simulink model "State_Flowc"  (R2017a)
settings: Solver=FixedStepDiscrete  StartTime=0.0  StopTime=inf  FixedStep=0.001  RelTol=1e-3  EnableMultiTasking=on
libraries: xpcethercatlib x31, simulink x4, simulink_extras x4, commutil2 x2
(part 2 of 2)

== matlab function State_Flowc/Movimento Braccia/Traiettorie figure/Quadrato ==
  data: xq output; yq output; t input; T input; h input; xq_p output; yq_p output
function [xq, yq, xq_p, yq_p] = Quadrato(t, T, h)
xv = 0.4;
xj = 0.1;
x1 = t/(0.5*T/4);
x2 = (t-0.5*T/4)/(T/4);
x3 = (t-1.5*T/4)/(T/4);
x4 = (t-2.5*T/4)/(T/4);
x5 = (t-3.5*T/4)/(0.5*T/4);
Ca = 1/((1-xv)*(xv-xj));
% Ca = 1/(xv*(1-xv));
% Cv = 1/(1-xv);


if t > 0 && t <= 0.5*T/4
  
  if ( x1 >= 0 && x1 < xj)            %acc crescente positiva
    f = Ca/xj*x1;
    F = (1/2)*Ca/xj*x1^2;
    G = (1/6)*Ca/xj*x1^3;
    J = Ca/xj;

  elseif (x1 >= xj && x1 < (xv-xj))   %acc costante positiva
    f = Ca;
    F = Ca*x1 - (1/2)*Ca*xj;
    G = (1/2)*Ca*x1^2 - (1/2)*Ca*xj*x1 + (1/6)*Ca*xj^2;
    J = 0;

  elseif( x1>= (xv-xj) && x1 < xv)    %acc decrescente positiva
    f = -Ca/xj*x1 + Ca*xv/xj;
    F = -(1/2)*Ca/xj*x1^2 + Ca/xj*xv*x1 - Ca*(xj + (1/2)/xj*xv^2 - xv);
    G = -(1/6)*Ca/xj*x1^3 + (1/2)*Ca/xj*xv*x1^2 - Ca*(xj + (1/2)/xj*xv^2 - xv)*x1 ...
        - (1/2)*Ca*xv^2  + (1/6)*Ca/xj*xv^3 + (1/2)*Ca*xv*xj;
    J = -Ca/xj;

  elseif( x1>= xv && x1 < (1-xv))     %acc costante nulla
    f = 0;
    F = Ca*(xv - xj);
    G = Ca*(xv - xj)*x1 - (1/2)*Ca*xv^2 + (1/2)*Ca*xv*xj;
    J = 0;
    
  elseif( x1>= (1-xv) && x1 < (1-xv+xj))   %acc decrescente negativa
    f = -Ca/xj*x1 + Ca/xj*(1-xv);
    F = -(1/2)*Ca/xj*x1^2 + Ca/xj*(1-xv)*x1 + Ca*(xv-xj) - (1/2)*Ca/xj*(1-xv)^2;
    G = -(1/6)*Ca/xj*x1^3 + (1/2)*Ca/xj*(1-xv)*x1^2 + Ca*(xv-xj)*x1 - (1/2)*Ca/xj*(1-xv)^2*x1 ...
        - (1/2)*Ca*xv^2 + (1/2)*Ca*xv*xj + (1/6)*Ca/xj*(1-xv)^3;
    J = -Ca/xj;
    
  elseif( x1>= (1-xv+xj) && x1 < (1-xj))   %acc costante negativa
    f = -Ca; 
    F = -Ca*x1 + Ca - (1/2)*Ca*xj;
    G = -(1/2)*Ca*x1^2 + Ca*x1 - (1/2)*Ca*xj*x1 + 1 - Ca*(-(1/2)*xj + (1/6)*xj^2 + (1/2));
    J = 0;
    
  elseif( x1>= (1-xj) && x1 <= 1)          %acc crescente negativa
    f = Ca/xj*(x1-1);
    F = (1/2)*Ca/xj*x1^2 - Ca/xj*x1 +(1/2)*Ca/xj;
    G = (1/6)*Ca/xj*x1^3 - (1/2)*Ca/xj*x1^2 +(1/2)*Ca/xj*x1 + 1 - (1/6)*Ca/xj;
    J = Ca/xj;
    
  else                                   %acc costante nulla
    f = 0;
    F = 0;
    G = 1;
    J = 0;
  end
    xq = G*h/2;
    xq_p = F*(h/2)/(T/4);
    yq = 0;
    yq_p = 0; 

elseif t > 0.5*T/4 && t <= 1.5*T/4
    Ca = 1/((1-xv)*(xv-xj));
% Cj = Ca/xj;
  
  if ( x2 >= 0 && x2 < xj)            %acc crescente positiva
    f = Ca/xj*x2;
    F = (1/2)*Ca/xj*x2^2;
    G = (1/6)*Ca/xj*x2^3;
    J = Ca/xj;

  elseif (x2 >= xj && x2 < (xv-xj))   %acc costante positiva
    f = Ca;
    F = Ca*x2 - (1/2)*Ca*xj;
    G = (1/2)*Ca*x2^2 - (1/2)*Ca*xj*x2 + (1/6)*Ca*xj^2;
    J = 0;

  elseif( x2>= (xv-xj) && x2 < xv)    %acc decrescente positiva
    f = -Ca/xj*x2 + Ca*xv/xj;
    F = -(1/2)*Ca/xj*x2^2 + Ca/xj*xv*x2 - Ca*(xj + (1/2)/xj*xv^2 - xv);
    G = -(1/6)*Ca/xj*x2^3 + (1/2)*Ca/xj*xv*x2^2 - Ca*(xj + (1/2)/xj*xv^2 - xv)*x2 ...
        - (1/2)*Ca*xv^2  + (1/6)*Ca/xj*xv^3 + (1/2)*Ca*xv*xj;
    J = -Ca/xj;

  elseif( x2>= xv && x2 < (1-xv))     %acc costante nulla
    f = 0;
    F = Ca*(xv - xj);
    G = Ca*(xv - xj)*x2 - (1/2)*Ca*xv^2 + (1/2)*Ca*xv*xj;
    J = 0;
    
  elseif( x2>= (1-xv) && x2 < (1-xv+xj))   %acc decrescente negativa
    f = -Ca/xj*x2 + Ca/xj*(1-xv);
    F = -(1/2)*Ca/xj*x2^2 + Ca/xj*(1-xv)*x2 + Ca*(xv-xj) - (1/2)*Ca/xj*(1-xv)^2;
    G = -(1/6)*Ca/xj*x2^3 + (1/2)*Ca/xj*(1-xv)*x2^2 + Ca*(xv-xj)*x2 - (1/2)*Ca/xj*(1-xv)^2*x2 ...
        - (1/2)*Ca*xv^2 + (1/2)*Ca*xv*xj + (1/6)*Ca/xj*(1-xv)^3;
    J = -Ca/xj;
    
  elseif( x2>= (1-xv+xj) && x2 < (1-xj))   %acc costante negativa
    f = -Ca; 
    F = -Ca*x2 + Ca - (1/2)*Ca*xj;
    G = -(1/2)*Ca*x2^2 + Ca*x2 - (1/2)*Ca*xj*x2 + 1 - Ca*(-(1/2)*xj + (1/6)*xj^2 + (1/2));
    J = 0;
    
  elseif( x2>= (1-xj) && x2 <= 1)          %acc crescente negativa
    f = Ca/xj*(x2-1);
    F = (1/2)*Ca/xj*x2^2 - Ca/xj*x2 +(1/2)*Ca/xj;
    G = (1/6)*Ca/xj*x2^3 - (1/2)*Ca/xj*x2^2 +(1/2)*Ca/xj*x2 + 1 - (1/6)*Ca/xj;
    J = Ca/xj;
    
  else                                   %acc costante nulla
    f = 0;
    F = 0;
    G = 1;
    J = 0;
  end
    xq = h/2;
    xq_p = 0;
    yq = -G*h; 
    yq_p = -F*h/(T/4); 

elseif t > 1.5*T/4 && t <= 2.5*T/4
     Ca = 1/((1-xv)*(xv-xj));
% Cj = Ca/xj;
  
  if ( x3 >= 0 && x3 < xj)            %acc crescente positiva
    f = Ca/xj*x3;
    F = (1/2)*Ca/xj*x3^2;
    G = (1/6)*Ca/xj*x3^3;
    J = Ca/xj;

  elseif (x3 >= xj && x3 < (xv-xj))   %acc costante positiva
    f = Ca;
    F = Ca*x3 - (1/2)*Ca*xj;
    G = (1/2)*Ca*x3^2 - (1/2)*Ca*xj*x3 + (1/6)*Ca*xj^2;
    J = 0;

  elseif( x3>= (xv-xj) && x3 < xv)    %acc decrescente positiva
    f = -Ca/xj*x3 + Ca*xv/xj;
    F = -(1/2)*Ca/xj*x3^2 + Ca/xj*xv*x3 - Ca*(xj + (1/2)/xj*xv^2 - xv);
    G = -(1/6)*Ca/xj*x3^3 + (1/2)*Ca/xj*xv*x3^2 - Ca*(xj + (1/2)/xj*xv^2 - xv)*x3 ...
        - (1/2)*Ca*xv^2  + (1/6)*Ca/xj*xv^3 + (1/2)*Ca*xv*xj;
    J = -Ca/xj;

  elseif( x3>= xv && x3 < (1-xv))     %acc costante nulla
    f = 0;
    F = Ca*(xv - xj);
    G = Ca*(xv - xj)*x3 - (1/2)*Ca*xv^2 + (1/2)*Ca*xv*xj;
    J = 0;
    
  elseif( x3>= (1-xv) && x3 < (1-xv+xj))   %acc decrescente negativa
    f = -Ca/xj*x3 + Ca/xj*(1-xv);
    F = -(1/2)*Ca/xj*x3^2 + Ca/xj*(1-xv)*x3 + Ca*(xv-xj) - (1/2)*Ca/xj*(1-xv)^2;
    G = -(1/6)*Ca/xj*x3^3 + (1/2)*Ca/xj*(1-xv)*x3^2 + Ca*(xv-xj)*x3 - (1/2)*Ca/xj*(1-xv)^2*x3 ...
        - (1/2)*Ca*xv^2 + (1/2)*Ca*xv*xj + (1/6)*Ca/xj*(1-xv)^3;
    J = -Ca/xj;
    
  elseif( x3>= (1-xv+xj) && x3 < (1-xj))   %acc costante negativa
    f = -Ca; 
    F = -Ca*x3 + Ca - (1/2)*Ca*xj;
    G = -(1/2)*Ca*x3^2 + Ca*x3 - (1/2)*Ca*xj*x3 + 1 - Ca*(-(1/2)*xj + (1/6)*xj^2 + (1/2));
    J = 0;
    
  elseif( x3>= (1-xj) && x3 <= 1)          %acc crescente negativa
    f = Ca/xj*(x3-1);
    F = (1/2)*Ca/xj*x3^2 - Ca/xj*x3 +(1/2)*Ca/xj;
    G = (1/6)*Ca/xj*x3^3 - (1/2)*Ca/xj*x3^2 +(1/2)*Ca/xj*x3 + 1 - (1/6)*Ca/xj;
    J = Ca/xj;
    
  else                                   %acc costante nulla
    f = 0;
    F = 0;
    G = 1;
    J = 0;
  end
    xq = h/2-G*h;
    xq_p = -F*h/(T/4);
    yq = -h; 
    yq_p = 0; 
 
elseif t > 2.5*T/4 && t <= 3.5*T/4
   Ca = 1/((1-xv)*(xv-xj));
% Cj = Ca/xj;
  
  if ( x4 >= 0 && x4 < xj)            %acc crescente positiva
    f = Ca/xj*x4;
    F = (1/2)*Ca/xj*x4^2;
    G = (1/6)*Ca/xj*x4^3;
    J = Ca/xj;

  elseif (x4 >= xj && x4 < (xv-xj))   %acc costante positiva
    f = Ca;
    F = Ca*x4 - (1/2)*Ca*xj;
    G = (1/2)*Ca*x4^2 - (1/2)*Ca*xj*x4 + (1/6)*Ca*xj^2;
    J = 0;

  elseif( x4>= (xv-xj) && x4 < xv)    %acc decrescente positiva
    f = -Ca/xj*x4 + Ca*xv/xj;
    F = -(1/2)*Ca/xj*x4^2 + Ca/xj*xv*x4 - Ca*(xj + (1/2)/xj*xv^2 - xv);
    G = -(1/6)*Ca/xj*x4^3 + (1/2)*Ca/xj*xv*x4^2 - Ca*(xj + (1/2)/xj*xv^2 - xv)*x4 ...
        - (1/2)*Ca*xv^2  + (1/6)*Ca/xj*xv^3 + (1/2)*Ca*xv*xj;
    J = -Ca/xj;

  elseif( x4>= xv && x4 < (1-xv))     %acc costante nulla
    f = 0;
    F = Ca*(xv - xj);
    G = Ca*(xv - xj)*x4 - (1/2)*Ca*xv^2 + (1/2)*Ca*xv*xj;
    J = 0;
    
  elseif( x4>= (1-xv) && x4 < (1-xv+xj))   %acc decrescente negativa
    f = -Ca/xj*x4 + Ca/xj*(1-xv);
    F = -(1/2)*Ca/xj*x4^2 + Ca/xj*(1-xv)*x4 + Ca*(xv-xj) - (1/2)*Ca/xj*(1-xv)^2;
    G = -(1/6)*Ca/xj*x4^3 + (1/2)*Ca/xj*(1-xv)*x4^2 + Ca*(xv-xj)*x4 - (1/2)*Ca/xj*(1-xv)^2*x4 ...
        - (1/2)*Ca*xv^2 + (1/2)*Ca*xv*xj + (1/6)*Ca/xj*(1-xv)^3;
    J = -Ca/xj;
    
  elseif( x4>= (1-xv+xj) && x4 < (1-xj))   %acc costante negativa
    f = -Ca; 
    F = -Ca*x4 + Ca - (1/2)*Ca*xj;
    G = -(1/2)*Ca*x4^2 + Ca*x4 - (1/2)*Ca*xj*x4 + 1 - Ca*(-(1/2)*xj + (1/6)*xj^2 + (1/2));
    J = 0;
    
  elseif( x4>= (1-xj) && x4 <= 1)          %acc crescente negativa
    f = Ca/xj*(x4-1);
    F = (1/2)*Ca/xj*x4^2 - Ca/xj*x4 +(1/2)*Ca/xj;
    G = (1/6)*Ca/xj*x4^3 - (1/2)*Ca/xj*x4^2 +(1/2)*Ca/xj*x4 + 1 - (1/6)*Ca/xj;
    J = Ca/xj;
    
  else                                   %acc costante nulla
    f = 0;
    F = 0;
    G = 1;
    J = 0;
  end
    xq = -h/2;
    xq_p = 0;
    yq = -h + G*h;
    yq_p = F*h/(T/4); 

elseif t > 3.5*T/4 && t <= 4*T/4
   Ca = 1/((1-xv)*(xv-xj));
% Cj = Ca/xj;
  
  if ( x5 >= 0 && x5 < xj)            %acc crescente positiva
    f = Ca/xj*x5;
    F = (1/2)*Ca/xj*x5^2;
    G = (1/6)*Ca/xj*x5^3;
    J = Ca/xj;

  elseif (x5 >= xj && x5 < (xv-xj))   %acc costante positiva
    f = Ca;
    F = Ca*x5 - (1/2)*Ca*xj;
    G = (1/2)*Ca*x5^2 - (1/2)*Ca*xj*x5 + (1/6)*Ca*xj^2;
    J = 0;

  elseif( x5>= (xv-xj) && x5 < xv)    %acc decrescente positiva
    f = -Ca/xj*x5 + Ca*xv/xj;
    F = -(1/2)*Ca/xj*x5^2 + Ca/xj*xv*x5 - Ca*(xj + (1/2)/xj*xv^2 - xv);
    G = -(1/6)*Ca/xj*x5^3 + (1/2)*Ca/xj*xv*x5^2 - Ca*(xj + (1/2)/xj*xv^2 - xv)*x5 ...
        - (1/2)*Ca*xv^2  + (1/6)*Ca/xj*xv^3 + (1/2)*Ca*xv*xj;
    J = -Ca/xj;

  elseif( x5>= xv && x5 < (1-xv))     %acc costante nulla
    f = 0;
    F = Ca*(xv - xj);
    G = Ca*(xv - xj)*x5 - (1/2)*Ca*xv^2 + (1/2)*Ca*xv*xj;
    J = 0;
    
  elseif( x5>= (1-xv) && x5 < (1-xv+xj))   %acc decrescente negativa
    f = -Ca/xj*x5 + Ca/xj*(1-xv);
    F = -(1/2)*Ca/xj*x5^2 + Ca/xj*(1-xv)*x5 + Ca*(xv-xj) - (1/2)*Ca/xj*(1-xv)^2;
    G = -(1/6)*Ca/xj*x5^3 + (1/2)*Ca/xj*(1-xv)*x5^2 + Ca*(xv-xj)*x5 - (1/2)*Ca/xj*(1-xv)^2*x5 ...
        - (1/2)*Ca*xv^2 + (1/2)*Ca*xv*xj + (1/6)*Ca/xj*(1-xv)^3;
    J = -Ca/xj;
    
  elseif( x5>= (1-xv+xj) && x5 < (1-xj))   %acc costante negativa
    f = -Ca; 
    F = -Ca*x5 + Ca - (1/2)*Ca*xj;
    G = -(1/2)*Ca*x5^2 + Ca*x5 - (1/2)*Ca*xj*x5 + 1 - Ca*(-(1/2)*xj + (1/6)*xj^2 + (1/2));
    J = 0;
    
  elseif( x5>= (1-xj) && x5 <= 1)          %acc crescente negativa
    f = Ca/xj*(x5-1);
    F = (1/2)*Ca/xj*x5^2 - Ca/xj*x5 +(1/2)*Ca/xj;
    G = (1/6)*Ca/xj*x5^3 - (1/2)*Ca/xj*x5^2 +(1/2)*Ca/xj*x5 + 1 - (1/6)*Ca/xj;
    J = Ca/xj;
    
  else                                   %acc costante nulla
    f = 0;
    F = 0;
    G = 1;
    J = 0;
  end
    xq = -h/2 + G*h/2;
    xq_p = F*h/2/(T/4);
    yq = 0
    yq_p = 0; 
else
xq = 0;
yq = 0;
xq_p = 0;
yq_p = 0; 
end

== matlab function State_Flowc/Sistema Braccia Linea/Velocita vite /Vel Asse A conv ==
  data: vA input; vel_A_conv output
function vel_A_conv = fcn(vA)
vel_A_conv = (vA)  *(2*pi)/163840/64;

== matlab function State_Flowc/Sistema Braccia Linea/Velocita vite /Vel Asse B conv ==
  data: p input; vel_B_conv output
function vel_B_conv = fcn(p)
vel_B_conv = p  *(2*pi)/163840/64;

== matlab function State_Flowc/Sistema Vite/Actual A/Posizione attuale Vite A/Asse A conv ==
  data: p input; pos_A_conv output
function pos_A_conv = fcn(p)
pos_A_conv = p * 0.02/(2*pi) * pi/2048/40;

== matlab function State_Flowc/Sistema Vite/Rifermento Asse A Vite ==
  data: t input; ldm_pos output; h input; T input; ldm_vel output
function [ldm_pos, ldm_vel] = fcn(t,h,T)

xv = 0.3;
 x = t/T;
Ca=1/(xv*(1-xv));
Cv = 1/(1-xv);

if( x>= 0 && x < xv)
    f = Ca;
    F = Ca*x;
    G= Ca*x^2/2;
elseif(x >= xv && x < (1-xv) )
    f = 0;
    F = Cv;
    G= Ca*xv^2/2 + Cv*(x-xv);
elseif( x >= (1-xv) && x <= 1 )
    f = -Ca;
    xloc = x-(1-xv);
    F = Cv -Ca*xloc;
    G= Ca*xv^2/2 + Cv*(1-2*xv) + Cv*xloc -Ca*xloc^2/2;
else
    f=0;
    F=0;
    G= Ca*xv^2/2 + Cv*(1-2*xv) + Cv*xv -Ca*xv^2/2;
end

ldm_pos = G*h;
ldm_vel = F*h/T;

== matlab function State_Flowc/LED Status/MATLAB Function ==
  data: u input; y output
function y = fcn(u)
if u == 2 ||u == 3
    y = 1;
else
    y = 0;
end

== matlab function State_Flowc/LED Status/MATLAB Function1 ==
  data: u input; y output
function y = fcn(u)
if u == 1 || u == 2 || u == 4
    y = 1;
else
    y = 0;
end

== matlab function State_Flowc/LED Status/MATLAB Function2 ==
  data: u input; y output
function y = fcn(u)
if u == 4 || u == 5
    y = 1;
else
    y = 0;
end

== matlab function State_Flowc/Sistema Vite/Asse B conv ==
  data: p input; pos_B_conv output
function pos_B_conv = fcn(p)
pos_B_conv = p * pi/2048/40;

== matlab function State_Flowc/Sistema Vite/Asse B ==
  data: t input; ldm_pos output; h input; T input; ldm_vel output
function [ldm_pos, ldm_vel] = fcn(t,h,T)

xv = 0.3;
 x = t/T;
Ca=1/(xv*(1-xv));
Cv = 1/(1-xv);

if( x>= 0 && x < xv)
    f = Ca;
    F = Ca*x;
    G= Ca*x^2/2;
elseif(x >= xv && x < (1-xv) )
    f = 0;
    F = Cv;
    G= Ca*xv^2/2 + Cv*(x-xv);
elseif( x >= (1-xv) && x <= 1 )
    f = -Ca;
    xloc = x-(1-xv);
    F = Cv -Ca*xloc;
    G= Ca*xv^2/2 + Cv*(1-2*xv) + Cv*xloc -Ca*xloc^2/2;
else
    f=0;
    F=0;
    G= Ca*xv^2/2 + Cv*(1-2*xv) + Cv*xv -Ca*xv^2/2;
end

ldm_pos = G*h;
ldm_vel = F*h/T;

== matlab function State_Flowc/Sistema Vite/Actual A/Posizione attuale Vite A/Asse B conv v ==
  data: p input; pos_B_conv_v output
function pos_B_conv_v = fcn(p)
pos_B_conv_v = p * 0.02/(2*pi) * pi/2048/40;

== matlab function State_Flowc/Sistema Vite/Velocita vite /Vel Asse A conv ==
  data: vA input; vel_A_conv output; vB input
function vel_A_conv = fcn(vA, vB)
vel_A_conv = (vA+vB) * 0.02/(2*pi) * pi/20480/40;

== matlab function State_Flowc/Sistema Vite/Velocita vite /Vel Asse B conv ==
  data: p input; vel_B_conv output
function vel_B_conv = fcn(p)
vel_B_conv = p  * pi/20480/40;

== stateflow chart State_Flowc/State flow robot ==
  settings: sampleTime=0.001
  state Step1
    entry:
    Bool = 0;
  state SetA
    entry:
    CoppiaA = 0;
    C1 = 0;
  state OffSet
    entry:
    CoppiaH = 0;
    CoppiaA = 0;
    CoppiaB = 0;
    OffA = posA;
    OffB = posB;
    OffA_0 = posA;
    OffB_0 = posB;
    Bool = 2;
    Luci = 3;
  state SetB1
    entry:
    CoppiaB = 0;
    C2 = 0;
  state Step2
    entry:
    CoppiaH = 0;
  state Discesa_Vite
    entry:
    OffA_vite = posA_vite;
    CoppiaH=700;
  state Controllo
    entry:
    OffA_vite = posA_vite;
    OffB_vite = posB_vite;
    Bool = 5;
    Luci = 5;
  state Traiettoria
    entry:
    OffT = Clock;
    Luci = 4;
    Bool = 4;
  state Coppie
    entry:
    OffA_0 = posA;
    OffB_0 = posB;
    CoppiaA = 1250;
    CoppiaB = 1250;
    CoppiaH = 0;
    Luci = 2;
  state Home
    entry:
    [CoppiaA, CoppiaB, CoppiaH] = Homing(fc, fcA, fcB);
    Bool = 1;
    conv =  (2*pi)/16384/64;
    conv_vite = 0.02/(2*pi) * pi/2048/40;
    Luci = 1;
    C1 = 1;
    C2 = 1;
  state SetB
    entry:
    CoppiaB = 0;
    C2 = 0;
  state SetA1
    entry:
    CoppiaA = 0;
    C1 = 0;
  state [CA,CB] = Mov1(posA,OffA,posB,OffB,OffT,Clock) [function] [commented out]
  state [CA,CB] = Mov(posA,OffA,posB,OffB,Clock, OffT, velA, velB) [function] [commented out]
  state [CA,CB,CH] = Homing(fc,fcA,fcB) [function]
  (default) -> Step1
  Discesa_Vite -> ? [order 1] : [posA_vite - OffA_vite >= 0.023/conv_vite]
  Coppie -> SetA [order 1] : [posA - OffA_0 >= 100*pi/180/conv]
  Step1 -> Home : [Status==1079]
  SetA -> SetB1 : [posB - OffB_0 >= 50*pi/180/conv]
  SetB1 -> Discesa_Vite : [C2 == 0]
  Home -> Step2 [order 2] : [fc==0]
  Step2 -> Coppie : [fcA == 1 && fcB==1]
  Traiettoria -> Controllo : after(10,sec)
  Discesa_Vite -> OffSet [order 1]
  OffSet -> Traiettoria
  SetA1 -> Discesa_Vite : [C1 == 0]
  SetB -> SetA1 : [posA - OffA_0 >= 100*pi/180/conv]
  Coppie -> SetB [order 2] : [posB - OffB_0 >= 50*pi/180/conv]
  Home -> Coppie [order 1] : [fcA==1 && fcB==1]
  data: posA function_input double size=1; CA function_output double size=1; CB function_output double size=1; OffA function_input double size=1; posB function_input double size=1; OffB function_input double size=1; OffT function_input double size=1; Clock function_input double size=1; CA function_output double size=1; CB function_output double size=1; posA function_input double size=1; OffA function_input double size=1; posB function_input double size=1; OffB function_input double size=1; Clock function_input double size=1; OffT function_input double size=1; velA function_input double size=1; velB function_input double size=1; fc function_input double size=1; CA function_output; CB function_output; CH function_output; fcA function_input double size=1; fcB function_input double size=1; Clock input; posA_vite input; posB_vite input; SampleTime constant double; Status input; fc input; posA input; posB input; Bool output; OffT output; CoppiaH output; OffA_vite output; OffB_vite output; OffA output; OffB output; CoppiaA output; CoppiaB output; fcA input; fcB input; conv local; Luci output; OffA_0 local; OffB_0 local; C1 local; C2 local; conv_vite local; velA input; velB input

== matlab function State_Flowc/Movimento Braccia/Cinematica Inversa ==
  data: x input; theta1 output; y input; theta2 output
function [theta1, theta2] = CinInversa(x, y)

d = 0.09; 
l = 0.25;

p = 2*d*l + 2*x*l;
e = 2*y*l;
f = x^2 + d^2 + y^2 + 2*x*d;
a = -2*d*l + 2*x*l;
b = +2*y*l;
c = x^2 + d^2 + y^2 - 2*x*d;



   theta1 = 2*atan2(e + sqrt(p^2 + e^2 -f^2), p +f);


   theta2 = 2*atan2(b - sqrt(a^2 + b^2 -c^2), a +c);
   if (theta2) < -deg2rad(200)
       theta2 = theta2 + 2*pi;
   end

== matlab function State_Flowc/Movimento Braccia/Posizione Braccio B/Asse B conv brac1 ==
  data: p input; pos_B_conv output
function pos_B_conv = fcn(p)
pos_B_conv = p * (2*pi)/16384/64;

== matlab function State_Flowc/State flow robot/Homing/MATLAB Function ==
  data: fc input; CA output; fcA input; fcB input; CB output; CH output
function [CA, CB, CH] = fcn(fc, fcA, fcB)

CA = -1500;
CB = -1500;
CH = -700;

if fc < 1
    CH = 0;
end
if fcA == 1
    CA = 0;
end
if fcB == 1
    CB = 0;
end

== matlab function State_Flowc/Out asse A Vite/Fungo/MATLAB Function ==
  data: now input; old input; y output
function y = fcn(now, old)
if old == 0 && now == 1
    y = 1;
else
    y = old;
end

== matlab function State_Flowc/Out asse B Vite/Fungo/MATLAB Function ==
  data: now input; old input; y output
function y = fcn(now, old)
if old == 0 && now == 1
    y = 1;
else
    y = old;
end

== matlab function State_Flowc/Out Asse A Braccia/Fungo/MATLAB Function ==
  data: now input; old input; y output
function y = fcn(now, old)
if old == 0 && now == 1
    y = 1;
else
    y = old;
end

== matlab function State_Flowc/Out Asse B Braccia/Fungo/MATLAB Function ==
  data: now input; old input; y output
function y = fcn(now, old)
if old == 0 && now == 1
    y = 1;
else
    y = old;
end

== matlab function State_Flowc/State flow robot/Mov/Cinematica Inversa ==
  data: x input; theta1 output; y input; theta2 output
function [theta1, theta2] = fcn(x, y)

d = 0.09; 
l = 0.25;

p = 2*d*l + 2*x*l;
e = 2*y*l;
f = x^2 + d^2 + y^2 + 2*x*d;
a = -2*d*l + 2*x*l;
b = +2*y*l;
c = x^2 + d^2 + y^2 - 2*x*d;



   theta1 = 2*atan2(e + sqrt(p^2 + e^2 -f^2), p +f);


   theta2 = 2*atan2(b - sqrt(a^2 + b^2 -c^2), a +c);
   if (theta2) < -deg2rad(200)
       theta2 = theta2 + 2*pi;
   end

== matlab function State_Flowc/State flow robot/Mov/Cinematica Inversa vel ==
  data: theta1 input; theta2 input; x input; y input; xp input; theta1_p output; yp input; theta2_p output
function [theta1_p, theta2_p] = fcn(theta1, theta2,x, y, xp, yp)

d = 0.09; 
l = 0.25;

N21 = -l*sin(theta1)*(x+d-l*cos(theta1)) + l*cos(theta1)*(y-l*sin(theta1));

N22 = -l*cos(theta2)*(y-l*sin(theta2))*(x+d-l*cos(theta1))/(x-d-l*cos(theta2)) + l*sin(theta2)*(x+d-l*cos(theta1));

D2 = y-l*sin(theta1) - (y-l*sin(theta2))*(x+d-l*cos(theta1))/(x-d-l*cos(theta2));

J21 = N21/D2;

J22 = N22/D2;

J11 = -(y-l*sin(theta2))/(x-d-l*cos(theta2))*(J21);

J12 = -(y-l*sin(theta2))/(x-d-l*cos(theta2))*(J22) -l*sin(theta2) + (y-l*sin(theta2))/(x-d-l*cos(theta2))*(l*cos(theta2));

J = [J11 J12; J21 J22];

theta_p = J^-1 * [xp; yp];
theta1_p = theta_p(1);
theta2_p = theta_p(2);

== matlab function State_Flowc/Velocita vite /Vel Asse A conv ==
  data: vA input; vel_A_conv output
function vel_A_conv = fcn(vA)
vel_A_conv = (vA)  *(2*pi)/163840/64;

== matlab function State_Flowc/Velocita vite /Vel Asse B conv ==
  data: p input; vel_B_conv output
function vel_B_conv = fcn(p)
vel_B_conv = p  *(2*pi)/163840/64;

== matlab function State_Flowc/State flow robot/Mov1/Asse A conv bracc ==
  data: p input; pos_A_conv output
function pos_A_conv = fcn(p)
pos_A_conv = p * (2*pi)/16384/64;

== matlab function State_Flowc/State flow robot/Mov1/Asse A conv bracc1 ==
  data: p input; pos_A_conv output
function pos_A_conv = fcn(p)
pos_A_conv = p * (2*pi)/16384/64;

== matlab function State_Flowc/State flow robot/Mov1/Ldm theta1 ==
  data: t input; theta1 output; T1 input
function theta1 = fcn(t,T1)
theta1 = T1(t*1000);
end

== matlab function State_Flowc/State flow robot/Mov1/Ldm theta2 ==
  data: t input; theta1 output; T1 input
function theta1 = fcn(t,T1)
theta1 = T1(t*1000);
end

== matlab function State_Flowc/State flow robot/Mov/x ==
  data: t input; ldm_pos output; h input; T input; ldm_vel output
function [ldm_pos, ldm_vel] = fcn(t,h,T)

xv = 0.3;
 x = t/T;
Ca=1/(xv*(1-xv));
Cv = 1/(1-xv);

if( x>= 0 && x < xv)
    f = Ca;
    F = Ca*x;
    G= Ca*x^2/2;
elseif(x >= xv && x < (1-xv) )
    f = 0;
    F = Cv;
    G= Ca*xv^2/2 + Cv*(x-xv);
elseif( x >= (1-xv) && x <= 1 )
    f = -Ca;
    xloc = x-(1-xv);
    F = Cv -Ca*xloc;
    G= Ca*xv^2/2 + Cv*(1-2*xv) + Cv*xloc -Ca*xloc^2/2;
else
    f=0;
    F=0;
    G= Ca*xv^2/2 + Cv*(1-2*xv) + Cv*xv -Ca*xv^2/2;
end

ldm_pos = G*h;
ldm_vel = F*h/T;

== matlab function State_Flowc/State flow robot/Mov/Asse A conv bracc2 ==
  data: p input; pos_A_conv output
function pos_A_conv = fcn(p)
pos_A_conv = p * (2*pi)/16384/64;

== matlab function State_Flowc/State flow robot/Mov/y ==
  data: t input; ldm_pos output; h input; T input; ldm_vel output
function [ldm_pos, ldm_vel] = fcn(t,h,T)

xv = 0.3;
 x = t/T;
Ca=1/(xv*(1-xv));
Cv = 1/(1-xv);

if( x>= 0 && x < xv)
    f = Ca;
    F = Ca*x;
    G= Ca*x^2/2;
elseif(x >= xv && x < (1-xv) )
    f = 0;
    F = Cv;
    G= Ca*xv^2/2 + Cv*(x-xv);
elseif( x >= (1-xv) && x <= 1 )
    f = -Ca;
    xloc = x-(1-xv);
    F = Cv -Ca*xloc;
    G= Ca*xv^2/2 + Cv*(1-2*xv) + Cv*xloc -Ca*xloc^2/2;
else
    f=0;
    F=0;
    G= Ca*xv^2/2 + Cv*(1-2*xv) + Cv*xv -Ca*xv^2/2;
end

ldm_pos = G*h;
ldm_vel = F*h/T;

== matlab function State_Flowc/State flow robot/Mov/Asse B conv brac ==
  data: p input; pos_B_conv output
function pos_B_conv = fcn(p)
pos_B_conv = p * (2*pi)/16384/64;

== matlab function State_Flowc/State flow robot/Mov/Cinematica Inversa1 ==
  data: theta1_0 input; x0 output; theta2_0 input; y0 output
function [x0, y0] = fcn(theta1_0, theta2_0)

d = 0.09; 
l = 0.25;

A = l^2*(sin(theta2_0)-sin(theta1_0))^2 + (-2*d -l*(cos(theta2_0)-cos(theta1_0)))^2;
B = -2*l^2*d*(sin(theta2_0)-sin(theta1_0))*(cos(theta2_0)+cos(theta1_0)) + ...
    l*(sin(theta2_0)-sin(theta1_0))*(-2*d -l*(cos(theta2_0)-cos(theta1_0)))*(-2*d -2*l*cos(theta2_0)) - ...
    2*l*sin(theta2_0)*(-2*d -l*(cos(theta2_0)-cos(theta1_0)))^2;
C = l^2*d^2*(cos(theta2_0)+cos(theta1_0))^2 -l*d*(cos(theta2_0)+cos(theta1_0))*(-2*d -l*(cos(theta2_0)-cos(theta1_0)))*(-2*d -2*l*cos(theta2_0)) + ...
    (d^2 + 2*d*l*cos(theta2_0))*(-2*d - l*(cos(theta2_0)-cos(theta1_0)))^2;

% Posizione Y end-effector
y0 = (-B + sqrt(B^2 - 4*A*C))/(2*A)
% Posizione X end-effector
x0 = (y0*l*(sin(theta2_0)-sin(theta1_0)) - l*d*(cos(theta2_0)+cos(theta1_0)))/(-2*d -l*(cos(theta2_0)-cos(theta1_0)))

== matlab function State_Flowc/Sistema Braccia Linea/Asse A conv bracc2 ==
  data: p input; pos_A_conv output
function pos_A_conv = fcn(p)
pos_A_conv = p * (2*pi)/16384/64;

== matlab function State_Flowc/Sistema Braccia Linea/Asse B conv brac1 ==
  data: p input; pos_B_conv output
function pos_B_conv = fcn(p)
pos_B_conv = p * (2*pi)/16384/64;

== matlab function State_Flowc/Sistema Braccia Linea/Cinematica Inversa ==
  data: x input; theta1 output; y input; theta2 output
function [theta1, theta2] = fcn(x, y)

d = 0.09; 
l = 0.25;

p = 2*d*l + 2*x*l;
e = 2*y*l;
f = x^2 + d^2 + y^2 + 2*x*d;
a = -2*d*l + 2*x*l;
b = +2*y*l;
c = x^2 + d^2 + y^2 - 2*x*d;



   theta1 = 2*atan2(e + sqrt(p^2 + e^2 -f^2), p +f);


   theta2 = 2*atan2(b - sqrt(a^2 + b^2 -c^2), a +c);
   if (theta2) < -deg2rad(200)
       theta2 = theta2 + 2*pi;
   end

== matlab function State_Flowc/Sistema Braccia Linea/Cinematica Inversa vel ==
  data: theta1 input; theta2 input; x input; y input; xp input; theta1_p output; yp input; theta2_p output
function [theta1_p, theta2_p] = fcn(theta1, theta2,x, y, xp, yp)

d = 0.09; 
l = 0.25;

N21 = -l*sin(theta1)*(x+d-l*cos(theta1)) + l*cos(theta1)*(y-l*sin(theta1));

N22 = -l*cos(theta2)*(y-l*sin(theta2))*(x+d-l*cos(theta1))/(x-d-l*cos(theta2)) + l*sin(theta2)*(x+d-l*cos(theta1));

D2 = y-l*sin(theta1) - (y-l*sin(theta2))*(x+d-l*cos(theta1))/(x-d-l*cos(theta2));

J21 = N21/D2;

J22 = N22/D2;

J11 = -(y-l*sin(theta2))/(x-d-l*cos(theta2))*(J21);

J12 = -(y-l*sin(theta2))/(x-d-l*cos(theta2))*(J22) -l*sin(theta2) + (y-l*sin(theta2))/(x-d-l*cos(theta2))*(l*cos(theta2));

J = [J11 J12; J21 J22];

theta_p = J^-1 * [xp; yp];
theta1_p = theta_p(1);
theta2_p = theta_p(2);

== matlab function State_Flowc/Sistema Braccia Linea/Cinematica Inversa1 ==
  data: theta1_0 input; x0 output; theta2_0 input; y0 output
function [x0, y0] = fcn(theta1_0, theta2_0)

d = 0.09; 
l = 0.25;

A = l^2*(sin(theta2_0)-sin(theta1_0))^2 + (-2*d -l*(cos(theta2_0)-cos(theta1_0)))^2;
B = -2*l^2*d*(sin(theta2_0)-sin(theta1_0))*(cos(theta2_0)+cos(theta1_0)) + ...
    l*(sin(theta2_0)-sin(theta1_0))*(-2*d -l*(cos(theta2_0)-cos(theta1_0)))*(-2*d -2*l*cos(theta2_0)) - ...
    2*l*sin(theta2_0)*(-2*d -l*(cos(theta2_0)-cos(theta1_0)))^2;
C = l^2*d^2*(cos(theta2_0)+cos(theta1_0))^2 -l*d*(cos(theta2_0)+cos(theta1_0))*(-2*d -l*(cos(theta2_0)-cos(theta1_0)))*(-2*d -2*l*cos(theta2_0)) + ...
    (d^2 + 2*d*l*cos(theta2_0))*(-2*d - l*(cos(theta2_0)-cos(theta1_0)))^2;

% Posizione Y end-effector
y0 = (-B + sqrt(B^2 - 4*A*C))/(2*A)
% Posizione X end-effector
x0 = (y0*l*(sin(theta2_0)-sin(theta1_0)) - l*d*(cos(theta2_0)+cos(theta1_0)))/(-2*d -l*(cos(theta2_0)-cos(theta1_0)))

== matlab function State_Flowc/Sistema Braccia Linea/x ==
  data: t input; ldm_pos output; h input; T input; ldm_vel output
function [ldm_pos, ldm_vel] = fcn(t,h,T)

xv = 0.3;
 x = t/T;
Ca=1/(xv*(1-xv));
Cv = 1/(1-xv);

if( x>= 0 && x < xv)
    f = Ca;
    F = Ca*x;
    G= Ca*x^2/2;
elseif(x >= xv && x < (1-xv) )
    f = 0;
    F = Cv;
    G= Ca*xv^2/2 + Cv*(x-xv);
elseif( x >= (1-xv) && x <= 1 )
    f = -Ca;
    xloc = x-(1-xv);
    F = Cv -Ca*xloc;
    G= Ca*xv^2/2 + Cv*(1-2*xv) + Cv*xloc -Ca*xloc^2/2;
else
    f=0;
    F=0;
    G= Ca*xv^2/2 + Cv*(1-2*xv) + Cv*xv -Ca*xv^2/2;
end

ldm_pos = G*h;
ldm_vel = F*h/T;

== matlab function State_Flowc/Sistema Braccia Linea/y ==
  data: t input; ldm_pos output; h input; T input; ldm_vel output
function [ldm_pos, ldm_vel] = fcn(t,h,T)

xv = 0.3;
 x = t/T;
Ca=1/(xv*(1-xv));
Cv = 1/(1-xv);

if( x>= 0 && x < xv)
    f = Ca;
    F = Ca*x;
    G= Ca*x^2/2;
elseif(x >= xv && x < (1-xv) )
    f = 0;
    F = Cv;
    G= Ca*xv^2/2 + Cv*(x-xv);
elseif( x >= (1-xv) && x <= 1 )
    f = -Ca;
    xloc = x-(1-xv);
    F = Cv -Ca*xloc;
    G= Ca*xv^2/2 + Cv*(1-2*xv) + Cv*xloc -Ca*xloc^2/2;
else
    f=0;
    F=0;
    G= 1;
end

ldm_pos = G*h;
ldm_vel = F*h/T;

== matlab function State_Flowc/Movimento Braccia/Posizione braccio A/Asse A conv brac ==
  data: p input; pos_A_conv output
function pos_A_conv = fcn(p)
pos_A_conv = p * (2*pi)/16384/64;

== matlab function State_Flowc/Movimento Braccia/Traiettorie figure/Cerchio ==
  data: x output; t input; y output; T input; h input; xp output; yp output
function [x, y,xp,yp] = Cerchio(t, T, h)
Y1 = linspace(0, -h, 1000*T/2);
Y2 = linspace(-h, 0, 1000*T/2);
if t > 0 && t <= T/2
    y = Y1(t*1000);
    x = sqrt(h^2 - y^2);
elseif t > T/2 && t <= T
    y = Y2((t-T/2)*1000);
    x = -sqrt(h^2 - y^2);
else
    x = 0;
    y = 0;
end

== matlab function State_Flowc/Movimento Braccia/Selettore ==
  data: x output; xq input; y output; yq input; xc input; yc input; select input
function [x, y] = fcn(xq, yq, xc, yc, select)
if select == 1
    x = xq;
    y = yq;
elseif select == 2
    x = xc;
    y = yc;
else
    x = 0;
    y = 0;
end

== matlab function State_Flowc/Movimento Braccia/Quadrato1 ==
  data: x output; t input; y output; T input; h input
function [x, y] = fcn(t, T, h)
X1 = linspace(0, h, 1000*T/4);
X2 = linspace(h, 0, 1000*T/4);
Y1 = linspace(0, -h, 1000*T/4);
Y2 = linspace(-h, 0, 1000*T/4);

if t > 0 && t <= T/4
    y = 0;
    x = X1(t*1000);
elseif t > T/4 && t <= 2*T/4
    x = h;
    y = Y1((t-T/4)*1000);
elseif t > 2*T/4 && t <= 3*T/4
    y = -h;
    x = X2((t-2*T/4)*1000);
elseif t > 3*T/4 && t <= 4*T/4
    x = 0;
    y = Y2((t-3*T/4)*1000);
else
x = 0;
y = 0;
end

== matlab function State_Flowc/Movimento Braccia/Cinematica Inversa vel ==
  data: theta1 input; theta2 input; x input; y input; xp input; theta1_p output; yp input; theta2_p output
function [theta1_p, theta2_p] = fcn(theta1, theta2,x, y, xp, yp)

d = 0.09; 
l = 0.25;

N21 = -l*sin(theta1)*(x+d-l*cos(theta1)) + l*cos(theta1)*(y-l*sin(theta1));

N22 = -l*cos(theta2)*(y-l*sin(theta2))*(x+d-l*cos(theta1))/(x-d-l*cos(theta2)) + l*sin(theta2)*(x+d-l*cos(theta1));

D2 = y-l*sin(theta1) - (y-l*sin(theta2))*(x+d-l*cos(theta1))/(x-d-l*cos(theta2));

J21 = N21/D2;

J22 = N22/D2;

J11 = -(y-l*sin(theta2))/(x-d-l*cos(theta2))*(J21);

J12 = -(y-l*sin(theta2))/(x-d-l*cos(theta2))*(J22) -l*sin(theta2) + (y-l*sin(theta2))/(x-d-l*cos(theta2))*(l*cos(theta2));

J = [J11 J12; J21 J22];

theta_p = J^-1 * [xp; yp];
theta1_p = theta_p(1);
theta2_p = theta_p(2);

== matlab function State_Flowc/Movimento Braccia/Coppie braccia/Velocita vite /Vel Asse B conv ==
  data: vB input; vel_B_conv output
function vel_B_conv = fcn(vB)
vel_B_conv = (vB)  *(2*pi)/163840/64;

== matlab function State_Flowc/Movimento Braccia/Coppie braccia/Velocita vite /Vel Asse A conv ==
  data: vA input; vel_A_conv output
function vel_A_conv = fcn(vA)
vel_A_conv = vA  *(2*pi)/163840/64;
